simulink model "radioteleskop"  (R2025b)
settings: Solver=ode4  StartTime=0.0  StopTime=6000  FixedStep=0.1  RelTol=1e-3
values from neighbouring files (symbols this model uses):
  Js = 2.16e6    (= 2160000)    [MdR_HA2_SoSe2026_Simulationen.m]
  kR = 0.1    [MdR_HA2_SoSe2026_Simulationen.m]
  M_W = 500    [MdR_HA2_SoSe2026_Simulationen.m]
  omega_0 = abs(lambda(1))    [MdR_HA1_SoSe26_Simulationen.m]    (also in MdR_HA2_SoSe2026_Simulationen.m = 0)
  phi_0 = deg2rad(25)    [MdR_HA1_SoSe26_Simulationen.m]    (also in MdR_HA2_SoSe2026_Simulationen.m = 0)
  t_d = 200    [MdR_HA2_SoSe2026_Simulationen.m]
  w_dot_0 = deg2rad(0.25) / 60    [MdR_HA2_SoSe2026_Simulationen.m]
libraries: simulink x1
settings Model: Creator=Asus  LastModifiedBy=Asus

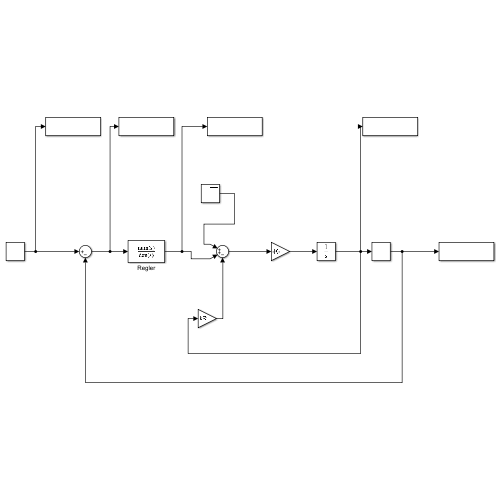
[thumbnail: Simulink's stored preview of the top-level diagram]
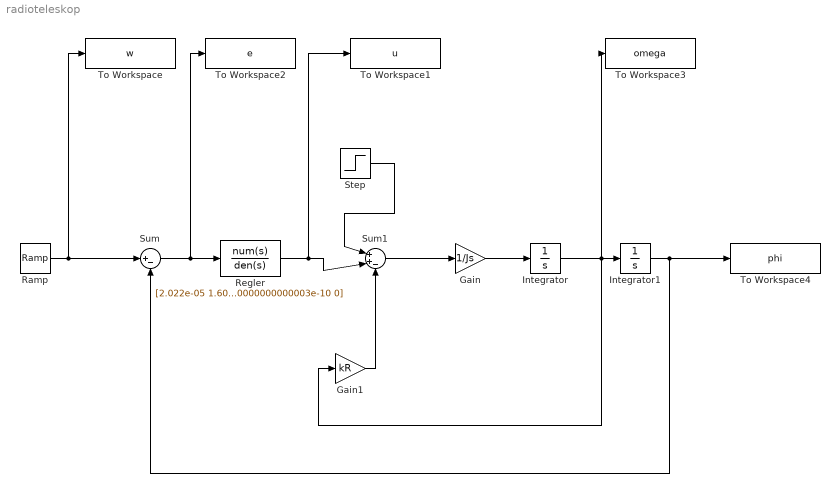
== system radioteleskop ==
  Gain : Gain  Gain=1/Js
  Gain1 : Gain  Gain=kR
  Integrator : Integrator  InitialCondition=omega_0  ContinuousStateAttributes='omega'
  Integrator1 : Integrator  InitialCondition=phi_0  ContinuousStateAttributes='phi'
  Ramp : simulink/Sources/Ramp  slope=w_dot_0  start=0  InitialOutput=0
  Regler : TransferFcn  Numerator=[2.022e-05 1.6089999999999999e-07 3.1999999999999998e-10]  Denominator=[4.6299999999999998e-08 9.3100000000000003e-09 4.6830000000000003e-10 0]  ParameterTunability=Unconstrained  ContinuousStateAttributes='REGLER'
  Step : Step  Time=t_d  After=M_W  SampleTime=0
  Sum : Sum  Inputs=|+-
  Sum1 : Sum  Inputs=|++-
  To Workspace : ToWorkspace  VariableName=w  SaveFormat=Timeseries  SampleTime=-1
  To Workspace1 : ToWorkspace  VariableName=u  SaveFormat=Timeseries  SampleTime=-1
  To Workspace2 : ToWorkspace  VariableName=e  SaveFormat=Timeseries  SampleTime=-1
  To Workspace3 : ToWorkspace  VariableName=omega  SaveFormat=Timeseries  SampleTime=-1
  To Workspace4 : ToWorkspace  VariableName=phi  SaveFormat=Timeseries  SampleTime=-1
  wires:
  Ramp/1 -> Sum/1, To Workspace/1
  Sum/1 -> Regler/1, To Workspace2/1
  Gain1/1 -> Sum1/3
  Sum1/1 -> Gain/1
  Gain/1 -> Integrator/1
  Integrator/1 -> Integrator1/1, Gain1/1, To Workspace3/1
  Integrator1/1 -> Sum/2, To Workspace4/1
  Regler/1 -> To Workspace1/1, Sum1/2
  Step/1 -> Sum1/1
